simulink model "three_H_bridge"  (R2022b)
settings: Solver=FixedStepAuto  StartTime=0.0  StopTime=0.1  FixedStep=1e-7  MaxStep=1e-6  RelTol=5e-6
InitFcn:
  | fs=5000;
  | t1=(1/(3*fs));%模块内的载波时延
  | t2=(2/(3*fs));
  | m=1;
libraries: spsMosfetLib x72, spsSeriesRLCBranchLib x48, spsVoltageMeasurementLib x19, simulink x18, spsDCVoltageSourceLib x18, sps_lib x1
(part 2 of 2)

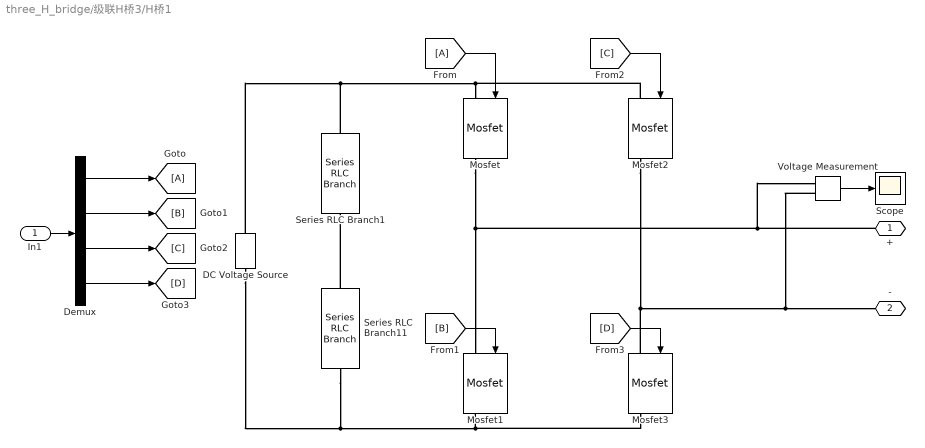
== system three_H_bridge/级联H桥3/H桥1 ==
  In1 : Inport
  DC Voltage Source : spsDCVoltageSourceLib/DC Voltage Source  Amplitude=650  Measurements=None
  Demux : Demux
  From : From
  Goto : Goto
  Mosfet{,1..3} (4 alike) : spsMosfetLib/Mosfet  Ron=0.1  Lon=0  Rd=0.01  Vfd=0  IC=0  Rs=1e5  Cs=inf  Measurements=on
  Scope : Scope
  Series RLC Branch1 : spsSeriesRLCBranchLib/Series RLC Branch  LConnTagsString=__new0  RConnTagsString=__new0  BranchType=RC  Resistance=0.001  Inductance=1e-3  SetiL0=off  InitialCurrent=0  Capacitance=60e-6  Setx0=off  InitialVoltage=0  Measurements=None
  Series RLC Branch11 : spsSeriesRLCBranchLib/Series RLC Branch  LConnTagsString=__new0  RConnTagsString=__new0  BranchType=RC  Resistance=0.001  Inductance=1e-3  SetiL0=off  InitialCurrent=0  Capacitance=60e-6  Setx0=off  InitialVoltage=0  Measurements=None
  Voltage Measurement : spsVoltageMeasurementLib/Voltage Measurement  PhasorSimulation=off  OutputType=Complex  PSBequivalent=0
  + : PMIOPort  Side=Right
  - : PMIOPort  Port=2  Side=Right
  wires:
  In1/1 -> Demux/1
  Demux/1 -> Goto/1
  Demux/2 -> [B]
  Demux/3 -> [C]
  Demux/4 -> [D]
  From/1 -> Mosfet/1
  [B] -> Mosfet1/1
  [C] -> Mosfet2/1
  [D] -> Mosfet3/1
  Voltage Measurement/1 -> Scope/1
  connections:
  DC Voltage Source/RConn1 -- Mosfet2/LConn1 -- Mosfet/LConn1 -- Series RLC Branch1/LConn1
  Mosfet2/RConn1 -- Mosfet3/LConn1 -- Voltage Measurement/LConn2 -- -/RConn1
  +/RConn1 -- Mosfet1/LConn1 -- Mosfet/RConn1 -- Voltage Measurement/LConn1
  DC Voltage Source/LConn1 -- Series RLC Branch11/RConn1 -- Mosfet3/RConn1 -- Mosfet1/RConn1
  Series RLC Branch11/LConn1 -- Series RLC Branch1/RConn1

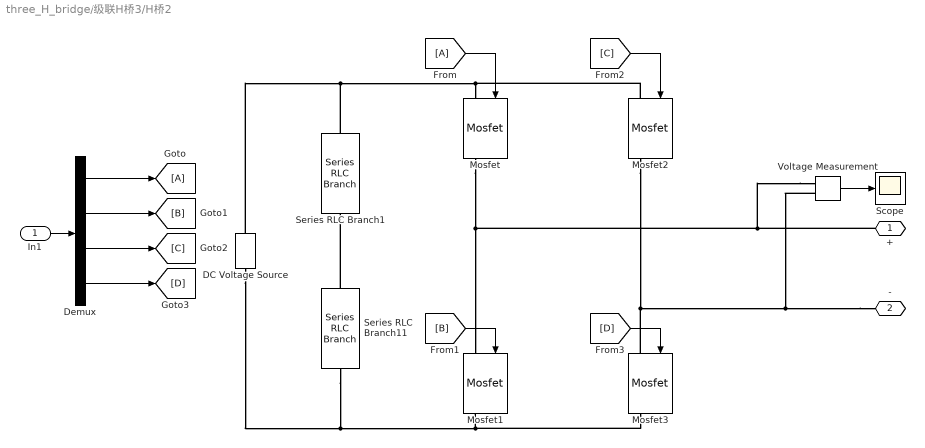
== system three_H_bridge/级联H桥3/H桥2 ==
  In1 : Inport
  DC Voltage Source : spsDCVoltageSourceLib/DC Voltage Source  Amplitude=650  Measurements=None
  Demux : Demux
  From : From
  Goto : Goto
  Mosfet{,1..3} (4 alike) : spsMosfetLib/Mosfet  Ron=0.1  Lon=0  Rd=0.01  Vfd=0  IC=0  Rs=1e5  Cs=inf  Measurements=on
  Scope : Scope
  Series RLC Branch1 : spsSeriesRLCBranchLib/Series RLC Branch  LConnTagsString=__new0  RConnTagsString=__new0  BranchType=RC  Resistance=0.001  Inductance=1e-3  SetiL0=off  InitialCurrent=0  Capacitance=60e-6  Setx0=off  InitialVoltage=0  Measurements=None
  Series RLC Branch11 : spsSeriesRLCBranchLib/Series RLC Branch  LConnTagsString=__new0  RConnTagsString=__new0  BranchType=RC  Resistance=0.001  Inductance=1e-3  SetiL0=off  InitialCurrent=0  Capacitance=60e-6  Setx0=off  InitialVoltage=0  Measurements=None
  Voltage Measurement : spsVoltageMeasurementLib/Voltage Measurement  PhasorSimulation=off  OutputType=Complex  PSBequivalent=0
  + : PMIOPort  Side=Right
  - : PMIOPort  Port=2  Side=Right
  wires:
  Voltage Measurement/1 -> Scope/1
  [D] -> Mosfet3/1
  [C] -> Mosfet2/1
  [B] -> Mosfet1/1
  From/1 -> Mosfet/1
  Demux/4 -> [D]
  Demux/3 -> [C]
  Demux/2 -> [B]
  Demux/1 -> Goto/1
  In1/1 -> Demux/1
  connections:
  Series RLC Branch11/LConn1 -- Series RLC Branch1/RConn1
  Mosfet1/RConn1 -- Mosfet3/RConn1 -- Series RLC Branch11/RConn1 -- DC Voltage Source/LConn1
  Voltage Measurement/LConn1 -- Mosfet/RConn1 -- Mosfet1/LConn1 -- +/RConn1
  -/RConn1 -- Voltage Measurement/LConn2 -- Mosfet3/LConn1 -- Mosfet2/RConn1
  Series RLC Branch1/LConn1 -- Mosfet/LConn1 -- Mosfet2/LConn1 -- DC Voltage Source/RConn1

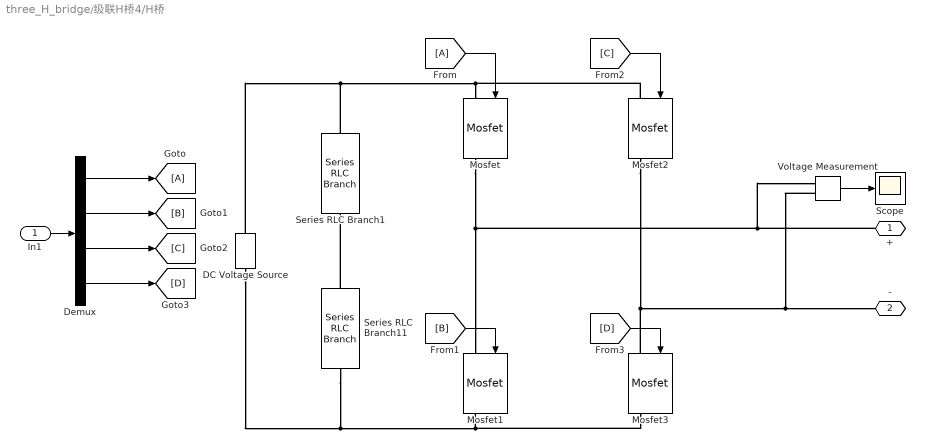
== system three_H_bridge/级联H桥4/H桥 ==
  In1 : Inport
  DC Voltage Source : spsDCVoltageSourceLib/DC Voltage Source  Amplitude=650  Measurements=None
  Demux : Demux
  From : From
  Goto : Goto
  Mosfet{,1..3} (4 alike) : spsMosfetLib/Mosfet  Ron=0.1  Lon=0  Rd=0.01  Vfd=0  IC=0  Rs=1e5  Cs=inf  Measurements=on
  Scope : Scope
  Series RLC Branch1 : spsSeriesRLCBranchLib/Series RLC Branch  LConnTagsString=__new0  RConnTagsString=__new0  BranchType=RC  Resistance=0.001  Inductance=1e-3  SetiL0=off  InitialCurrent=0  Capacitance=60e-6  Setx0=off  InitialVoltage=0  Measurements=None
  Series RLC Branch11 : spsSeriesRLCBranchLib/Series RLC Branch  LConnTagsString=__new0  RConnTagsString=__new0  BranchType=RC  Resistance=0.001  Inductance=1e-3  SetiL0=off  InitialCurrent=0  Capacitance=60e-6  Setx0=off  InitialVoltage=0  Measurements=None
  Voltage Measurement : spsVoltageMeasurementLib/Voltage Measurement  PhasorSimulation=off  OutputType=Complex  PSBequivalent=0
  + : PMIOPort  Side=Right
  - : PMIOPort  Port=2  Side=Right
  wires:
  In1/1 -> Demux/1
  Demux/1 -> Goto/1
  Demux/2 -> [B]
  Demux/3 -> [C]
  Demux/4 -> [D]
  From/1 -> Mosfet/1
  [B] -> Mosfet1/1
  [C] -> Mosfet2/1
  [D] -> Mosfet3/1
  Voltage Measurement/1 -> Scope/1
  connections:
  DC Voltage Source/RConn1 -- Mosfet2/LConn1 -- Mosfet/LConn1 -- Series RLC Branch1/LConn1
  Mosfet2/RConn1 -- Mosfet3/LConn1 -- Voltage Measurement/LConn2 -- -/RConn1
  +/RConn1 -- Mosfet1/LConn1 -- Mosfet/RConn1 -- Voltage Measurement/LConn1
  DC Voltage Source/LConn1 -- Series RLC Branch11/RConn1 -- Mosfet3/RConn1 -- Mosfet1/RConn1
  Series RLC Branch11/LConn1 -- Series RLC Branch1/RConn1

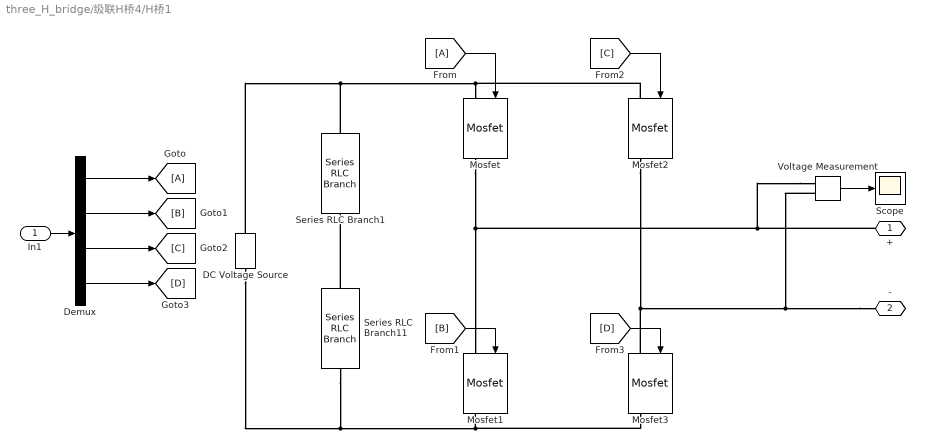
== system three_H_bridge/级联H桥4/H桥1 ==
  In1 : Inport
  DC Voltage Source : spsDCVoltageSourceLib/DC Voltage Source  Amplitude=650  Measurements=None
  Demux : Demux
  From : From
  Goto : Goto
  Mosfet{,1..3} (4 alike) : spsMosfetLib/Mosfet  Ron=0.1  Lon=0  Rd=0.01  Vfd=0  IC=0  Rs=1e5  Cs=inf  Measurements=on
  Scope : Scope
  Series RLC Branch1 : spsSeriesRLCBranchLib/Series RLC Branch  LConnTagsString=__new0  RConnTagsString=__new0  BranchType=RC  Resistance=0.001  Inductance=1e-3  SetiL0=off  InitialCurrent=0  Capacitance=60e-6  Setx0=off  InitialVoltage=0  Measurements=None
  Series RLC Branch11 : spsSeriesRLCBranchLib/Series RLC Branch  LConnTagsString=__new0  RConnTagsString=__new0  BranchType=RC  Resistance=0.001  Inductance=1e-3  SetiL0=off  InitialCurrent=0  Capacitance=60e-6  Setx0=off  InitialVoltage=0  Measurements=None
  Voltage Measurement : spsVoltageMeasurementLib/Voltage Measurement  PhasorSimulation=off  OutputType=Complex  PSBequivalent=0
  + : PMIOPort  Side=Right
  - : PMIOPort  Port=2  Side=Right
  wires:
  Voltage Measurement/1 -> Scope/1
  [D] -> Mosfet3/1
  [C] -> Mosfet2/1
  [B] -> Mosfet1/1
  From/1 -> Mosfet/1
  Demux/4 -> [D]
  Demux/3 -> [C]
  Demux/2 -> [B]
  Demux/1 -> Goto/1
  In1/1 -> Demux/1
  connections:
  Series RLC Branch11/LConn1 -- Series RLC Branch1/RConn1
  Mosfet1/RConn1 -- Mosfet3/RConn1 -- Series RLC Branch11/RConn1 -- DC Voltage Source/LConn1
  Voltage Measurement/LConn1 -- Mosfet/RConn1 -- Mosfet1/LConn1 -- +/RConn1
  -/RConn1 -- Voltage Measurement/LConn2 -- Mosfet3/LConn1 -- Mosfet2/RConn1
  Series RLC Branch1/LConn1 -- Mosfet/LConn1 -- Mosfet2/LConn1 -- DC Voltage Source/RConn1

== system three_H_bridge/级联H桥4/H桥2 ==
  In1 : Inport
  DC Voltage Source : spsDCVoltageSourceLib/DC Voltage Source  Amplitude=650  Measurements=None
  Demux : Demux
  From : From
  Goto : Goto
  Mosfet{,1..3} (4 alike) : spsMosfetLib/Mosfet  Ron=0.1  Lon=0  Rd=0.01  Vfd=0  IC=0  Rs=1e5  Cs=inf  Measurements=on
  Scope : Scope
  Series RLC Branch1 : spsSeriesRLCBranchLib/Series RLC Branch  LConnTagsString=__new0  RConnTagsString=__new0  BranchType=RC  Resistance=0.001  Inductance=1e-3  SetiL0=off  InitialCurrent=0  Capacitance=60e-6  Setx0=off  InitialVoltage=0  Measurements=None
  Series RLC Branch11 : spsSeriesRLCBranchLib/Series RLC Branch  LConnTagsString=__new0  RConnTagsString=__new0  BranchType=RC  Resistance=0.001  Inductance=1e-3  SetiL0=off  InitialCurrent=0  Capacitance=60e-6  Setx0=off  InitialVoltage=0  Measurements=None
  Voltage Measurement : spsVoltageMeasurementLib/Voltage Measurement  PhasorSimulation=off  OutputType=Complex  PSBequivalent=0
  + : PMIOPort  Side=Right
  - : PMIOPort  Port=2  Side=Right
  wires:
  In1/1 -> Demux/1
  Demux/1 -> Goto/1
  Demux/2 -> [B]
  Demux/3 -> [C]
  Demux/4 -> [D]
  From/1 -> Mosfet/1
  [B] -> Mosfet1/1
  [C] -> Mosfet2/1
  [D] -> Mosfet3/1
  Voltage Measurement/1 -> Scope/1
  connections:
  DC Voltage Source/RConn1 -- Mosfet2/LConn1 -- Mosfet/LConn1 -- Series RLC Branch1/LConn1
  Mosfet2/RConn1 -- Mosfet3/LConn1 -- Voltage Measurement/LConn2 -- -/RConn1
  +/RConn1 -- Mosfet1/LConn1 -- Mosfet/RConn1 -- Voltage Measurement/LConn1
  DC Voltage Source/LConn1 -- Series RLC Branch11/RConn1 -- Mosfet3/RConn1 -- Mosfet1/RConn1
  Series RLC Branch11/LConn1 -- Series RLC Branch1/RConn1

== system three_H_bridge/级联H桥5/H桥 ==
  In1 : Inport
  DC Voltage Source : spsDCVoltageSourceLib/DC Voltage Source  Amplitude=650  Measurements=None
  Demux : Demux
  From : From
  Goto : Goto
  Mosfet{,1..3} (4 alike) : spsMosfetLib/Mosfet  Ron=0.1  Lon=0  Rd=0.01  Vfd=0  IC=0  Rs=1e5  Cs=inf  Measurements=on
  Scope : Scope
  Series RLC Branch1 : spsSeriesRLCBranchLib/Series RLC Branch  LConnTagsString=__new0  RConnTagsString=__new0  BranchType=RC  Resistance=0.001  Inductance=1e-3  SetiL0=off  InitialCurrent=0  Capacitance=60e-6  Setx0=off  InitialVoltage=0  Measurements=None
  Series RLC Branch11 : spsSeriesRLCBranchLib/Series RLC Branch  LConnTagsString=__new0  RConnTagsString=__new0  BranchType=RC  Resistance=0.001  Inductance=1e-3  SetiL0=off  InitialCurrent=0  Capacitance=60e-6  Setx0=off  InitialVoltage=0  Measurements=None
  Voltage Measurement : spsVoltageMeasurementLib/Voltage Measurement  PhasorSimulation=off  OutputType=Complex  PSBequivalent=0
  + : PMIOPort  Side=Right
  - : PMIOPort  Port=2  Side=Right
  wires:
  Voltage Measurement/1 -> Scope/1
  [D] -> Mosfet3/1
  [C] -> Mosfet2/1
  [B] -> Mosfet1/1
  From/1 -> Mosfet/1
  Demux/4 -> [D]
  Demux/3 -> [C]
  Demux/2 -> [B]
  Demux/1 -> Goto/1
  In1/1 -> Demux/1
  connections:
  Series RLC Branch11/LConn1 -- Series RLC Branch1/RConn1
  Mosfet1/RConn1 -- Mosfet3/RConn1 -- Series RLC Branch11/RConn1 -- DC Voltage Source/LConn1
  Voltage Measurement/LConn1 -- Mosfet/RConn1 -- Mosfet1/LConn1 -- +/RConn1
  -/RConn1 -- Voltage Measurement/LConn2 -- Mosfet3/LConn1 -- Mosfet2/RConn1
  Series RLC Branch1/LConn1 -- Mosfet/LConn1 -- Mosfet2/LConn1 -- DC Voltage Source/RConn1

== system three_H_bridge/级联H桥5/H桥1 ==
  In1 : Inport
  DC Voltage Source : spsDCVoltageSourceLib/DC Voltage Source  Amplitude=650  Measurements=None
  Demux : Demux
  From : From
  Goto : Goto
  Mosfet{,1..3} (4 alike) : spsMosfetLib/Mosfet  Ron=0.1  Lon=0  Rd=0.01  Vfd=0  IC=0  Rs=1e5  Cs=inf  Measurements=on
  Scope : Scope
  Series RLC Branch1 : spsSeriesRLCBranchLib/Series RLC Branch  LConnTagsString=__new0  RConnTagsString=__new0  BranchType=RC  Resistance=0.001  Inductance=1e-3  SetiL0=off  InitialCurrent=0  Capacitance=60e-6  Setx0=off  InitialVoltage=0  Measurements=None
  Series RLC Branch11 : spsSeriesRLCBranchLib/Series RLC Branch  LConnTagsString=__new0  RConnTagsString=__new0  BranchType=RC  Resistance=0.001  Inductance=1e-3  SetiL0=off  InitialCurrent=0  Capacitance=60e-6  Setx0=off  InitialVoltage=0  Measurements=None
  Voltage Measurement : spsVoltageMeasurementLib/Voltage Measurement  PhasorSimulation=off  OutputType=Complex  PSBequivalent=0
  + : PMIOPort  Side=Right
  - : PMIOPort  Port=2  Side=Right
  wires:
  In1/1 -> Demux/1
  Demux/1 -> Goto/1
  Demux/2 -> [B]
  Demux/3 -> [C]
  Demux/4 -> [D]
  From/1 -> Mosfet/1
  [B] -> Mosfet1/1
  [C] -> Mosfet2/1
  [D] -> Mosfet3/1
  Voltage Measurement/1 -> Scope/1
  connections:
  DC Voltage Source/RConn1 -- Mosfet2/LConn1 -- Mosfet/LConn1 -- Series RLC Branch1/LConn1
  Mosfet2/RConn1 -- Mosfet3/LConn1 -- Voltage Measurement/LConn2 -- -/RConn1
  +/RConn1 -- Mosfet1/LConn1 -- Mosfet/RConn1 -- Voltage Measurement/LConn1
  DC Voltage Source/LConn1 -- Series RLC Branch11/RConn1 -- Mosfet3/RConn1 -- Mosfet1/RConn1
  Series RLC Branch11/LConn1 -- Series RLC Branch1/RConn1

== system three_H_bridge/级联H桥5/H桥2 ==
  In1 : Inport
  DC Voltage Source : spsDCVoltageSourceLib/DC Voltage Source  Amplitude=650  Measurements=None
  Demux : Demux
  From : From
  Goto : Goto
  Mosfet{,1..3} (4 alike) : spsMosfetLib/Mosfet  Ron=0.1  Lon=0  Rd=0.01  Vfd=0  IC=0  Rs=1e5  Cs=inf  Measurements=on
  Scope : Scope
  Series RLC Branch1 : spsSeriesRLCBranchLib/Series RLC Branch  LConnTagsString=__new0  RConnTagsString=__new0  BranchType=RC  Resistance=0.001  Inductance=1e-3  SetiL0=off  InitialCurrent=0  Capacitance=60e-6  Setx0=off  InitialVoltage=0  Measurements=None
  Series RLC Branch11 : spsSeriesRLCBranchLib/Series RLC Branch  LConnTagsString=__new0  RConnTagsString=__new0  BranchType=RC  Resistance=0.001  Inductance=1e-3  SetiL0=off  InitialCurrent=0  Capacitance=60e-6  Setx0=off  InitialVoltage=0  Measurements=None
  Voltage Measurement : spsVoltageMeasurementLib/Voltage Measurement  PhasorSimulation=off  OutputType=Complex  PSBequivalent=0
  + : PMIOPort  Side=Right
  - : PMIOPort  Port=2  Side=Right
  wires:
  Voltage Measurement/1 -> Scope/1
  [D] -> Mosfet3/1
  [C] -> Mosfet2/1
  [B] -> Mosfet1/1
  From/1 -> Mosfet/1
  Demux/4 -> [D]
  Demux/3 -> [C]
  Demux/2 -> [B]
  Demux/1 -> Goto/1
  In1/1 -> Demux/1
  connections:
  Series RLC Branch11/LConn1 -- Series RLC Branch1/RConn1
  Mosfet1/RConn1 -- Mosfet3/RConn1 -- Series RLC Branch11/RConn1 -- DC Voltage Source/LConn1
  Voltage Measurement/LConn1 -- Mosfet/RConn1 -- Mosfet1/LConn1 -- +/RConn1
  -/RConn1 -- Voltage Measurement/LConn2 -- Mosfet3/LConn1 -- Mosfet2/RConn1
  Series RLC Branch1/LConn1 -- Mosfet/LConn1 -- Mosfet2/LConn1 -- DC Voltage Source/RConn1

== system three_H_bridge/级联H桥6/H桥 ==
  In1 : Inport
  DC Voltage Source : spsDCVoltageSourceLib/DC Voltage Source  Amplitude=650  Measurements=None
  Demux : Demux
  From : From
  Goto : Goto
  Mosfet{,1..3} (4 alike) : spsMosfetLib/Mosfet  Ron=0.1  Lon=0  Rd=0.01  Vfd=0  IC=0  Rs=1e5  Cs=inf  Measurements=on
  Scope : Scope
  Series RLC Branch1 : spsSeriesRLCBranchLib/Series RLC Branch  LConnTagsString=__new0  RConnTagsString=__new0  BranchType=RC  Resistance=0.001  Inductance=1e-3  SetiL0=off  InitialCurrent=0  Capacitance=60e-6  Setx0=off  InitialVoltage=0  Measurements=None
  Series RLC Branch11 : spsSeriesRLCBranchLib/Series RLC Branch  LConnTagsString=__new0  RConnTagsString=__new0  BranchType=RC  Resistance=0.001  Inductance=1e-3  SetiL0=off  InitialCurrent=0  Capacitance=60e-6  Setx0=off  InitialVoltage=0  Measurements=None
  Voltage Measurement : spsVoltageMeasurementLib/Voltage Measurement  PhasorSimulation=off  OutputType=Complex  PSBequivalent=0
  + : PMIOPort  Side=Right
  - : PMIOPort  Port=2  Side=Right
  wires:
  In1/1 -> Demux/1
  Demux/1 -> Goto/1
  Demux/2 -> [B]
  Demux/3 -> [C]
  Demux/4 -> [D]
  From/1 -> Mosfet/1
  [B] -> Mosfet1/1
  [C] -> Mosfet2/1
  [D] -> Mosfet3/1
  Voltage Measurement/1 -> Scope/1
  connections:
  DC Voltage Source/RConn1 -- Mosfet2/LConn1 -- Mosfet/LConn1 -- Series RLC Branch1/LConn1
  Mosfet2/RConn1 -- Mosfet3/LConn1 -- Voltage Measurement/LConn2 -- -/RConn1
  +/RConn1 -- Mosfet1/LConn1 -- Mosfet/RConn1 -- Voltage Measurement/LConn1
  DC Voltage Source/LConn1 -- Series RLC Branch11/RConn1 -- Mosfet3/RConn1 -- Mosfet1/RConn1
  Series RLC Branch11/LConn1 -- Series RLC Branch1/RConn1

== system three_H_bridge/级联H桥6/H桥1 ==
  In1 : Inport
  DC Voltage Source : spsDCVoltageSourceLib/DC Voltage Source  Amplitude=650  Measurements=None
  Demux : Demux
  From : From
  Goto : Goto
  Mosfet{,1..3} (4 alike) : spsMosfetLib/Mosfet  Ron=0.1  Lon=0  Rd=0.01  Vfd=0  IC=0  Rs=1e5  Cs=inf  Measurements=on
  Scope : Scope
  Series RLC Branch1 : spsSeriesRLCBranchLib/Series RLC Branch  LConnTagsString=__new0  RConnTagsString=__new0  BranchType=RC  Resistance=0.001  Inductance=1e-3  SetiL0=off  InitialCurrent=0  Capacitance=60e-6  Setx0=off  InitialVoltage=0  Measurements=None
  Series RLC Branch11 : spsSeriesRLCBranchLib/Series RLC Branch  LConnTagsString=__new0  RConnTagsString=__new0  BranchType=RC  Resistance=0.001  Inductance=1e-3  SetiL0=off  InitialCurrent=0  Capacitance=60e-6  Setx0=off  InitialVoltage=0  Measurements=None
  Voltage Measurement : spsVoltageMeasurementLib/Voltage Measurement  PhasorSimulation=off  OutputType=Complex  PSBequivalent=0
  + : PMIOPort  Side=Right
  - : PMIOPort  Port=2  Side=Right
  wires:
  Voltage Measurement/1 -> Scope/1
  [D] -> Mosfet3/1
  [C] -> Mosfet2/1
  [B] -> Mosfet1/1
  From/1 -> Mosfet/1
  Demux/4 -> [D]
  Demux/3 -> [C]
  Demux/2 -> [B]
  Demux/1 -> Goto/1
  In1/1 -> Demux/1
  connections:
  Series RLC Branch11/LConn1 -- Series RLC Branch1/RConn1
  Mosfet1/RConn1 -- Mosfet3/RConn1 -- Series RLC Branch11/RConn1 -- DC Voltage Source/LConn1
  Voltage Measurement/LConn1 -- Mosfet/RConn1 -- Mosfet1/LConn1 -- +/RConn1
  -/RConn1 -- Voltage Measurement/LConn2 -- Mosfet3/LConn1 -- Mosfet2/RConn1
  Series RLC Branch1/LConn1 -- Mosfet/LConn1 -- Mosfet2/LConn1 -- DC Voltage Source/RConn1

== system three_H_bridge/级联H桥6/H桥2 ==
  In1 : Inport
  DC Voltage Source : spsDCVoltageSourceLib/DC Voltage Source  Amplitude=650  Measurements=None
  Demux : Demux
  From : From
  Goto : Goto
  Mosfet{,1..3} (4 alike) : spsMosfetLib/Mosfet  Ron=0.1  Lon=0  Rd=0.01  Vfd=0  IC=0  Rs=1e5  Cs=inf  Measurements=on
  Scope : Scope
  Series RLC Branch1 : spsSeriesRLCBranchLib/Series RLC Branch  LConnTagsString=__new0  RConnTagsString=__new0  BranchType=RC  Resistance=0.001  Inductance=1e-3  SetiL0=off  InitialCurrent=0  Capacitance=60e-6  Setx0=off  InitialVoltage=0  Measurements=None
  Series RLC Branch11 : spsSeriesRLCBranchLib/Series RLC Branch  LConnTagsString=__new0  RConnTagsString=__new0  BranchType=RC  Resistance=0.001  Inductance=1e-3  SetiL0=off  InitialCurrent=0  Capacitance=60e-6  Setx0=off  InitialVoltage=0  Measurements=None
  Voltage Measurement : spsVoltageMeasurementLib/Voltage Measurement  PhasorSimulation=off  OutputType=Complex  PSBequivalent=0
  + : PMIOPort  Side=Right
  - : PMIOPort  Port=2  Side=Right
  wires:
  In1/1 -> Demux/1
  Demux/1 -> Goto/1
  Demux/2 -> [B]
  Demux/3 -> [C]
  Demux/4 -> [D]
  From/1 -> Mosfet/1
  [B] -> Mosfet1/1
  [C] -> Mosfet2/1
  [D] -> Mosfet3/1
  Voltage Measurement/1 -> Scope/1
  connections:
  DC Voltage Source/RConn1 -- Mosfet2/LConn1 -- Mosfet/LConn1 -- Series RLC Branch1/LConn1
  Mosfet2/RConn1 -- Mosfet3/LConn1 -- Voltage Measurement/LConn2 -- -/RConn1
  +/RConn1 -- Mosfet1/LConn1 -- Mosfet/RConn1 -- Voltage Measurement/LConn1
  DC Voltage Source/LConn1 -- Series RLC Branch11/RConn1 -- Mosfet3/RConn1 -- Mosfet1/RConn1
  Series RLC Branch11/LConn1 -- Series RLC Branch1/RConn1
